simulink model "Ex3_Antenna_Array_Integration"  (R2025b)
settings: Solver=FixedStepDiscrete  StartTime=0.0  StopTime=0.01  RelTol=1e-3
InitFcn:
  | fc     = 2.4e9;
  | c      = physconst('Lightspeed');
  | lambda = freq2wavelen(fc,c);
undefined symbols (not defined in the file or in its folder): physconst
libraries: dspstat3 x2, phasedtxrxlib x1
settings Model: Creator=galberti  LastModifiedBy=galberti

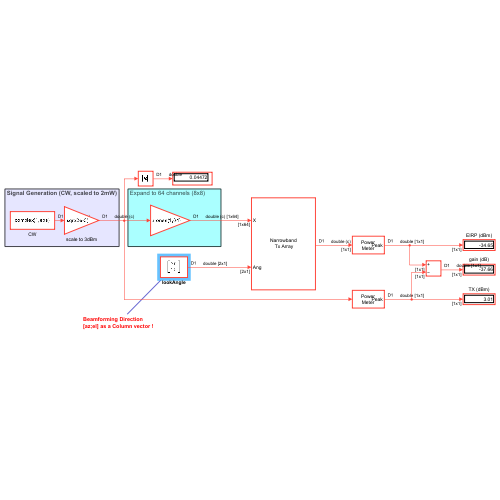
[thumbnail: Simulink's stored preview of the top-level diagram]
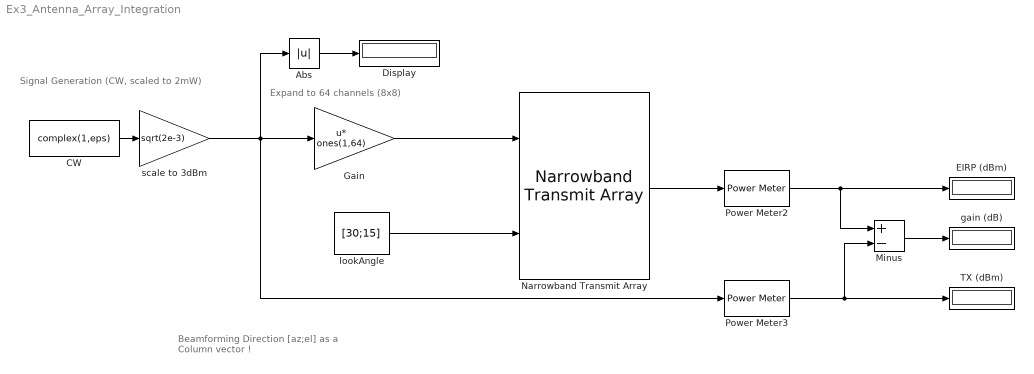
== system Ex3_Antenna_Array_Integration ==
  note: Beamforming Direction
      | [az;el] as a Column vector !
  note: Expand to 64 channels (8x8)
  note: Signal Generation (CW, scaled to 2mW)
  Abs : Abs  SaturateOnIntegerOverflow=off
  CW : Constant  Value=complex(1,eps)  SampleTime=1e-6
  Display : Display
  EIRP (dBm) : Display
  Gain : Gain  Gain=ones(1,64)  Multiplication=Matrix(u*K)
  Minus : Sum  Inputs=+-
  Narrowband Transmit Array : phasedtxrxlib/Narrowband Transmit Array  PropagationSpeed=physconst( 'LightSpeed' )  OperatingFrequency=2.4e9  CombineRadiatedSignals=on  SensorGainMeasure=dBi  Polarization=None  WeightsInputPort=off  SimulateUsing=Interpreted execution  Sensor=phased.URA(Size=[8,8],ElementSpacing=[ 0.5, 0.5 ] .*lambda,ArrayNormal='x',Element=phased.IsotropicAntennaElement())
  Power Meter2 : dspstat3/Power Meter  Measurement=Peak power  ReferenceLoad=1  OutputPowerUnits=dBm  WindowLength=256  OverlapLength=255  AllowArbitraryInputLength=off  ComputeCCDF=off  PowerRange=50  PowerResolution=0.1  CCDFOutput=Relative power (dB above average power)  ProbabilityVector=[ 10; 1; 0.1; 0.01; 0.001; 0.0001 ]  RelativePowerVector=[ 0; 3; 6; 9; 12 ]  ResetPort=off  SimulateUsing=Interpreted execution
      settings: LibrarySourceBlock=commutil2/Power Meter
  Power Meter3 : dspstat3/Power Meter  Measurement=Peak power  ReferenceLoad=1  OutputPowerUnits=dBm  WindowLength=256  OverlapLength=255  AllowArbitraryInputLength=off  ComputeCCDF=off  PowerRange=50  PowerResolution=0.1  CCDFOutput=Relative power (dB above average power)  ProbabilityVector=[ 10; 1; 0.1; 0.01; 0.001; 0.0001 ]  RelativePowerVector=[ 0; 3; 6; 9; 12 ]  ResetPort=off  SimulateUsing=Interpreted execution
      settings: LibrarySourceBlock=commutil2/Power Meter
  TX (dBm) : Display
  gain (dB) : Display
  lookAngle : Constant  Value=[30;15]  VectorParams1D=off  SampleTime=1e-6
  scale to 3dBm : Gain  Gain=sqrt(2e-3)
  wires:
  lookAngle/1 -> Narrowband Transmit Array/2
  Narrowband Transmit Array/1 -> Power Meter2/1
  Power Meter2/1 -> EIRP (dBm)/1, Minus/1
  CW/1 -> scale to 3dBm/1
  scale to 3dBm/1 -> Abs/1, Power Meter3/1, Gain/1
  Power Meter3/1 -> TX (dBm)/1, Minus/2
  Gain/1 -> Narrowband Transmit Array/1
  Minus/1 -> gain (dB)/1
  Abs/1 -> Display/1
